simulink subsystem "NonlinearPendulum"  (R2025b)
settings: Solver=VariableStepAuto  StartTime=0.0  StopTime=10.0  RelTol=1e-3
model mask{b=0.86, g=9.81, l=0.1, theta0=pi/4, dtheta0=0}
  mask prompts: b "Friction Coefficient"; g "Gravity"; l "Rod Length"; theta0 "Initial Position"; dtheta0 "Initial Velocity"
settings Model: Creator=alvaro  LastModifiedBy=alvaro

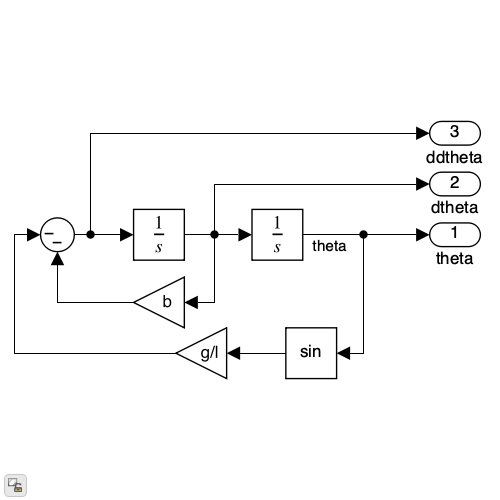
[thumbnail: Simulink's stored preview of the top-level diagram]
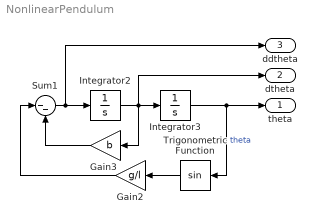
== system NonlinearPendulum ==
  Gain2 : Gain  Gain=g/l
  Gain3 : Gain  Gain=b
  Integrator2 : Integrator  InitialCondition=dtheta0
  Integrator3 : Integrator  InitialCondition=theta0
  Sum1 : Sum  Inputs=|--
  Trigonometric Function : Trigonometry
  theta : Outport
  dtheta : Outport  Port=2
  ddtheta : Outport  Port=3
  wires:
  Gain2/1 -> Sum1/1
  Sum1/1 -> Integrator2/1, ddtheta/1
  Integrator2/1 -> Integrator3/1, Gain3/1, dtheta/1
  Gain3/1 -> Sum1/2
  Integrator3/1 -> theta/1, Trigonometric Function/1  "theta"
  Trigonometric Function/1 -> Gain2/1
